simulink model "svpwm"  (R2024a)
settings: Solver=VariableStepAuto  StartTime=0.0  StopTime=0.2  RelTol=1e-3
libraries: simulink x3, spsThreePhaseProgrammableGeneratorLib x1
settings Model: Creator=SUNNY  LastModifiedBy=SUNNY

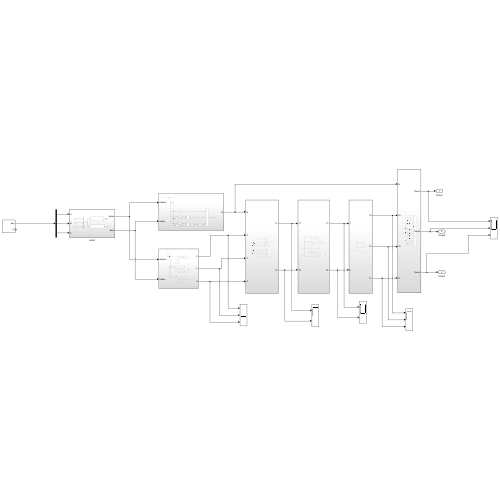
[thumbnail: Simulink's stored preview of the top-level diagram]
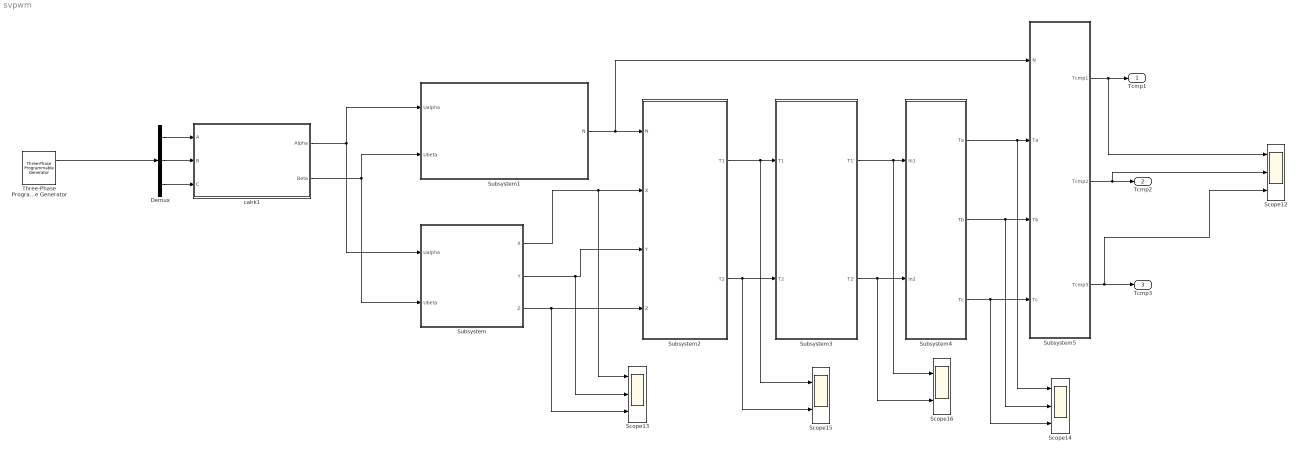
== system svpwm ==
  Demux : Demux  Outputs=3
  Scope12 : Scope  NumInputPorts=3
  Scope13 : Scope  NumInputPorts=3
  Scope14 : Scope  NumInputPorts=3
  Scope15 : Scope  NumInputPorts=2
  Scope16 : Scope  NumInputPorts=2
  Subsystem : Subsystem
  Subsystem1 : Subsystem
  Subsystem2 : Subsystem
  Subsystem3 : Subsystem
  Subsystem4 : Subsystem
  Subsystem5 : Subsystem
  Three-Phase Programmable Generator : spsThreePhaseProgrammableGeneratorLib/Three-Phase Programmable Generator  Par_Vps=[100, 0, 50]  VariationEntity=None  VariationType=Ramp  VariationStep=-0.5  VariationRate=10  VariationMag=0.3  VariationFreq=2  Par_Timing_Variation="[0.2  1.2]"  SinglePhase=on  Yampli=[1 0.2 1.2 1.0]  Xtime=[0 0.1 0.15 0.2]  HarmonicGeneration=off  Par_HarmoA="[3  5  -25 0]"  Par_HarmoB="[5  10  35  2]"  Par_Timing_Harmo="[ 0.05  99]"  Ts=1e-5
      settings: LibrarySourceBlock=|
      | sps_lib/Sources/Signal Generator Sources/Three-Phase
      | Programmable
      | Generator
  calrk1 : Subsystem
  Tcmp1 : Outport
  Tcmp2 : Outport  Port=2
  Tcmp3 : Outport  Port=3
  wires:
  calrk1/2(Beta) -> Subsystem/2(Ubeta), Subsystem1/2(Ubeta)
  Subsystem3/1(T1') -> Scope16/1, Subsystem4/1(In1)
  Three-Phase Programmable Generator/1 -> Demux/1
  Demux/3 -> calrk1/3(C)
  Subsystem2/1(T1) -> Scope15/1, Subsystem3/1(T1)
  Subsystem2/2(T2) -> Scope15/2, Subsystem3/2(T2)
  calrk1/1(Alpha) -> Subsystem/1(Ualpha), Subsystem1/1(Ualpha)
  Subsystem3/2(T2') -> Scope16/2, Subsystem4/2(In2)
  Subsystem5/2(Tcmp2) -> Scope12/2, Tcmp2/1
  Subsystem4/1(Ta) -> Scope14/1, Subsystem5/2(Ta)
  Subsystem4/3(Tc) -> Scope14/3, Subsystem5/4(Tc)
  Subsystem5/3(Tcmp3) -> Scope12/3, Tcmp3/1
  Demux/2 -> calrk1/2(B)
  Demux/1 -> calrk1/1(A)
  Subsystem5/1(Tcmp1) -> Scope12/1, Tcmp1/1
  Subsystem4/2(Tb) -> Scope14/2, Subsystem5/3(Tb)
  Subsystem/2(Y) -> Scope13/2, Subsystem2/3(Y)
  Subsystem/3(Z) -> Scope13/3, Subsystem2/4(Z)
  Subsystem1/1(N) -> Subsystem5/1(N), Subsystem2/1(N)
  Subsystem/1(X) -> Scope13/1, Subsystem2/2(X)

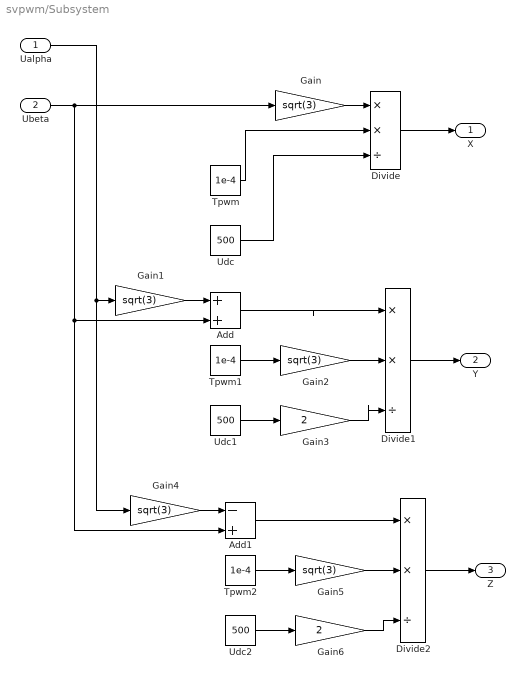
== system svpwm/Subsystem ==
  Ualpha : Inport
  Ubeta : Inport  Port=2
  Add : Sum
  Add1 : Sum  Inputs=-+
  Divide : Product  Inputs=**/
  Divide1 : Product  Inputs=**/
  Divide2 : Product  Inputs=**/
  Gain{,1..2,4..5} (5 alike) : Gain  Gain=sqrt(3)
  Gain3 : Gain  Gain=2
  Gain6 : Gain  Gain=2
  Tpwm : Constant  Value=1e-4
  Tpwm1 : Constant  Value=1e-4
  Tpwm2 : Constant  Value=1e-4
  Udc : Constant  Value=500
  Udc1 : Constant  Value=500
  Udc2 : Constant  Value=500
  X : Outport
  Y : Outport  Port=2
  Z : Outport  Port=3
  wires:
  Divide2/1 -> Z/1
  Gain2/1 -> Divide1/2
  Udc1/1 -> Gain3/1
  Add/1 -> Divide1/1
  Ubeta/1 -> Add1/2, Add/2, Gain/1
  Tpwm/1 -> Divide/2
  Gain1/1 -> Add/1
  Gain4/1 -> Add1/1
  Gain5/1 -> Divide2/2
  Udc/1 -> Divide/3
  Ualpha/1 -> Gain4/1, Gain1/1
  Gain/1 -> Divide/1
  Divide/1 -> X/1
  Tpwm1/1 -> Gain2/1
  Gain3/1 -> Divide1/3
  Udc2/1 -> Gain6/1
  Tpwm2/1 -> Gain5/1
  Add1/1 -> Divide2/1
  Gain6/1 -> Divide2/3
  Divide1/1 -> Y/1

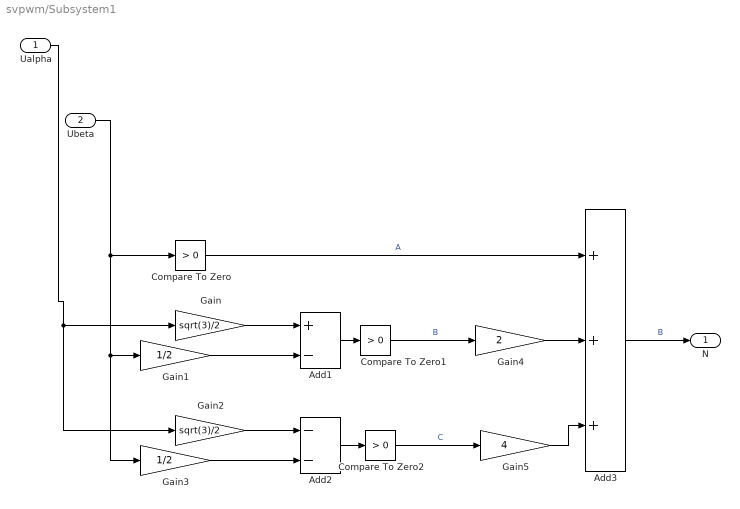
== system svpwm/Subsystem1 ==
  Ualpha : Inport
  Ubeta : Inport  Port=2
  Add1 : Sum  Inputs=+-
  Add2 : Sum  Inputs=--
  Add3 : Sum  Inputs=+++
  Compare To Zero : simulink/Logic and Bit Operations/Compare To Zero  relop=>  OutDataTypeStr=boolean
  Compare To Zero1 : simulink/Logic and Bit Operations/Compare To Zero  relop=>  OutDataTypeStr=boolean
  Compare To Zero2 : simulink/Logic and Bit Operations/Compare To Zero  relop=>  OutDataTypeStr=boolean
  Gain : Gain  Gain=sqrt(3)/2
  Gain1 : Gain  Gain=1/2
  Gain2 : Gain  Gain=sqrt(3)/2
  Gain3 : Gain  Gain=1/2
  Gain4 : Gain  Gain=2
  Gain5 : Gain  Gain=4
  N : Outport
  wires:
  Ubeta/1 -> Gain3/1, Gain1/1, Compare To Zero/1
  Gain3/1 -> Add2/2
  Gain2/1 -> Add2/1
  Ualpha/1 -> Gain2/1, Gain/1
  Compare To Zero/1 -> Add3/1  "A"
  Gain/1 -> Add1/1
  Gain1/1 -> Add1/2
  Add3/1 -> N/1  "B"
  Gain5/1 -> Add3/3
  Gain4/1 -> Add3/2
  Add2/1 -> Compare To Zero2/1
  Add1/1 -> Compare To Zero1/1
  Compare To Zero1/1 -> Gain4/1  "B"
  Compare To Zero2/1 -> Gain5/1  "C"

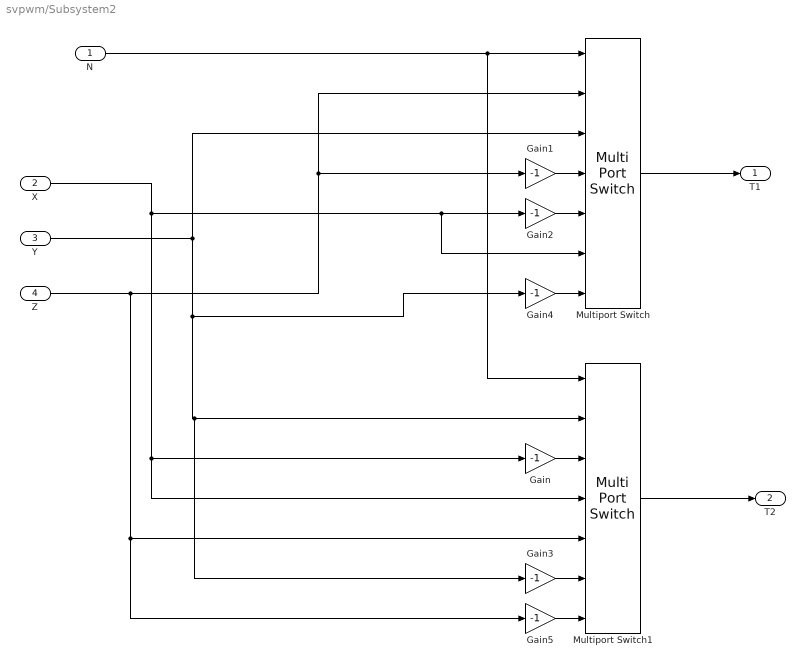
== system svpwm/Subsystem2 ==
  N : Inport
  X : Inport  Port=2
  Y : Inport  Port=3
  Z : Inport  Port=4
  Gain{,1..5} (6 alike) : Gain  Gain=-1
  Multiport Switch : MultiPortSwitch  Inputs=6  SaturateOnIntegerOverflow=off  InputSameDT=off
  Multiport Switch1 : MultiPortSwitch  Inputs=6  SaturateOnIntegerOverflow=off  InputSameDT=off
  T1 : Outport
  T2 : Outport  Port=2
  wires:
  Gain2/1 -> Multiport Switch/5
  Gain4/1 -> Multiport Switch/7
  Y/1 -> Gain4/1, Gain3/1, Multiport Switch1/2, Multiport Switch/3
  Multiport Switch/1 -> T1/1
  Z/1 -> Gain5/1, Multiport Switch1/5, Gain1/1, Multiport Switch/2
  Gain3/1 -> Multiport Switch1/6
  X/1 -> Multiport Switch/6, Gain2/1, Multiport Switch1/4, Gain/1
  Gain1/1 -> Multiport Switch/4
  N/1 -> Multiport Switch/1, Multiport Switch1/1
  Gain/1 -> Multiport Switch1/3
  Multiport Switch1/1 -> T2/1
  Gain5/1 -> Multiport Switch1/7

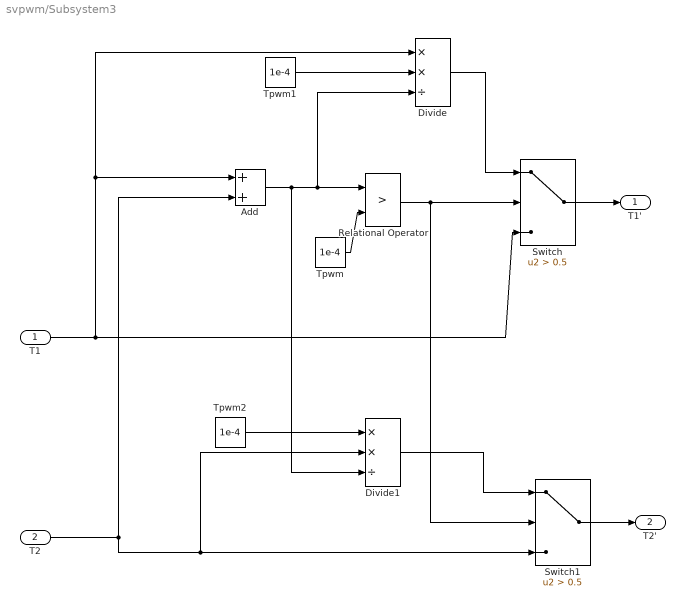
== system svpwm/Subsystem3 ==
  T1 : Inport
  T2 : Inport  Port=2
  Add : Sum
  Divide : Product  Inputs=**/
  Divide1 : Product  Inputs=**/
  Relational Operator : RelationalOperator  Operator=>  OutDataTypeStr=boolean  RndMeth=Simplest  InputSameDT=off
  Switch : Switch  Criteria=u2 > Threshold  Threshold=0.5  SaturateOnIntegerOverflow=off  InputSameDT=off
  Switch1 : Switch  Criteria=u2 > Threshold  Threshold=0.5  SaturateOnIntegerOverflow=off  InputSameDT=off
  Tpwm : Constant  Value=1e-4
  Tpwm1 : Constant  Value=1e-4
  Tpwm2 : Constant  Value=1e-4
  T1' : Outport
  T2' : Outport  Port=2
  wires:
  Switch/1 -> T1'/1
  T1/1 -> Switch/3, Divide/1, Add/1
  Add/1 -> Divide1/3, Divide/3, Relational Operator/1
  Tpwm/1 -> Relational Operator/2
  T2/1 -> Switch1/3, Divide1/2, Add/2
  Relational Operator/1 -> Switch1/2, Switch/2
  Switch1/1 -> T2'/1
  Tpwm1/1 -> Divide/2
  Tpwm2/1 -> Divide1/1
  Divide1/1 -> Switch1/1
  Divide/1 -> Switch/1

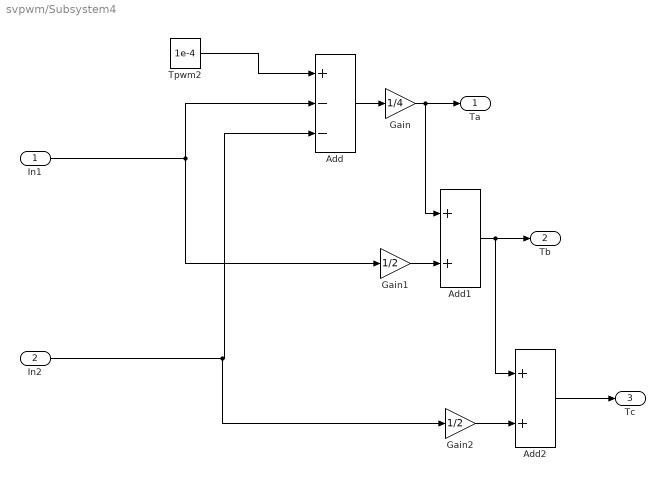
== system svpwm/Subsystem4 ==
  In1 : Inport
  In2 : Inport  Port=2
  Add : Sum  Inputs=+--
  Add1 : Sum
  Add2 : Sum
  Gain : Gain  Gain=1/4
  Gain1 : Gain  Gain=1/2
  Gain2 : Gain  Gain=1/2
  Tpwm2 : Constant  Value=1e-4
  Ta : Outport
  Tb : Outport  Port=2
  Tc : Outport  Port=3
  wires:
  Add/1 -> Gain/1
  In1/1 -> Gain1/1, Add/2
  Gain/1 -> Ta/1, Add1/1
  Add2/1 -> Tc/1
  In2/1 -> Gain2/1, Add/3
  Gain1/1 -> Add1/2
  Tpwm2/1 -> Add/1
  Gain2/1 -> Add2/2
  Add1/1 -> Tb/1, Add2/1

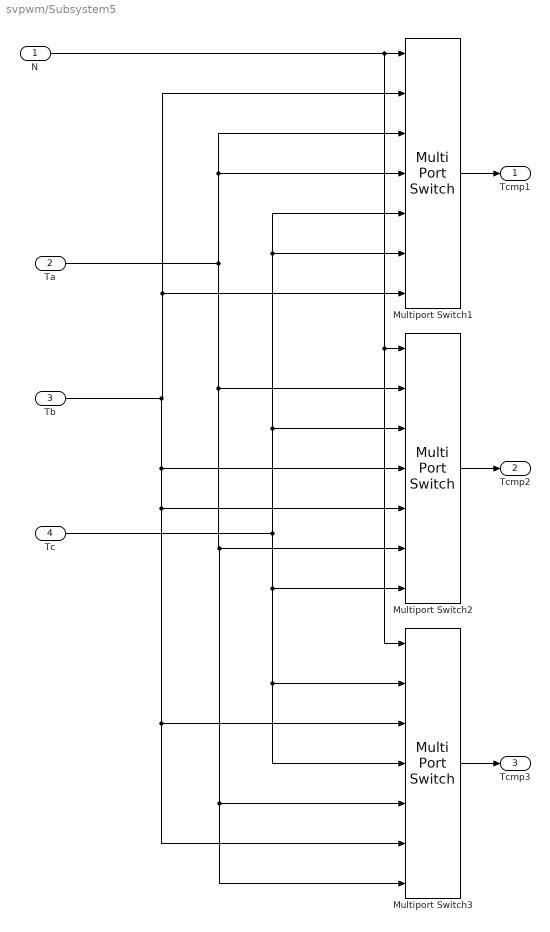
== system svpwm/Subsystem5 ==
  N : Inport
  Ta : Inport  Port=2
  Tb : Inport  Port=3
  Tc : Inport  Port=4
  Multiport Switch1 : MultiPortSwitch  Inputs=6  SaturateOnIntegerOverflow=off  InputSameDT=off
  Multiport Switch2 : MultiPortSwitch  Inputs=6  SaturateOnIntegerOverflow=off  InputSameDT=off
  Multiport Switch3 : MultiPortSwitch  Inputs=6  SaturateOnIntegerOverflow=off  InputSameDT=off
  Tcmp1 : Outport
  Tcmp2 : Outport  Port=2
  Tcmp3 : Outport  Port=3
  wires:
  Multiport Switch2/1 -> Tcmp2/1
  N/1 -> Multiport Switch3/1, Multiport Switch2/1, Multiport Switch1/1
  Ta/1 -> Multiport Switch3/7, Multiport Switch3/5, Multiport Switch2/6, Multiport Switch2/2, Multiport Switch1/4, Multiport Switch1/3
  Multiport Switch1/1 -> Tcmp1/1
  Tb/1 -> Multiport Switch3/6, Multiport Switch3/3, Multiport Switch2/5, Multiport Switch2/4, Multiport Switch1/7, Multiport Switch1/2
  Multiport Switch3/1 -> Tcmp3/1
  Tc/1 -> Multiport Switch2/3, Multiport Switch1/6, Multiport Switch1/5, Multiport Switch2/7, Multiport Switch3/4, Multiport Switch3/2

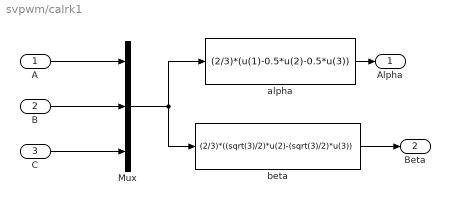
== system svpwm/calrk1 ==
  A : Inport
  B : Inport  Port=2
  C : Inport  Port=3
  Mux : Mux  Inputs=3
  alpha : Fcn  Expr=(2/3)*(u(1)-0.5*u(2)-0.5*u(3))
  beta : Fcn  Expr=(2/3)*((sqrt(3)/2)*u(2)-(sqrt(3)/2)*u(3))
  Alpha : Outport
  Beta : Outport  Port=2
  wires:
  beta/1 -> Beta/1
  alpha/1 -> Alpha/1
  A/1 -> Mux/1
  B/1 -> Mux/2
  C/1 -> Mux/3
  Mux/1 -> beta/1, alpha/1
